simulink model "W05_2_idx_memory"  (R2024b)
settings: Solver=ode4  StartTime=0.0  StopTime=20  FixedStep=Ts_ctrl  RelTol=1e-3
values from neighbouring files (symbols this model uses):
  Ts_ctrl = 0.05    [W05_setup.m]    (also in W07_setup.m)
settings Model: Creator=admin  LastModifiedBy=admin

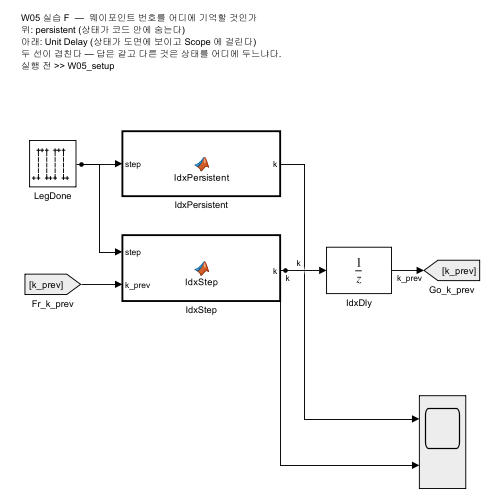
[thumbnail: Simulink's stored preview of the top-level diagram]
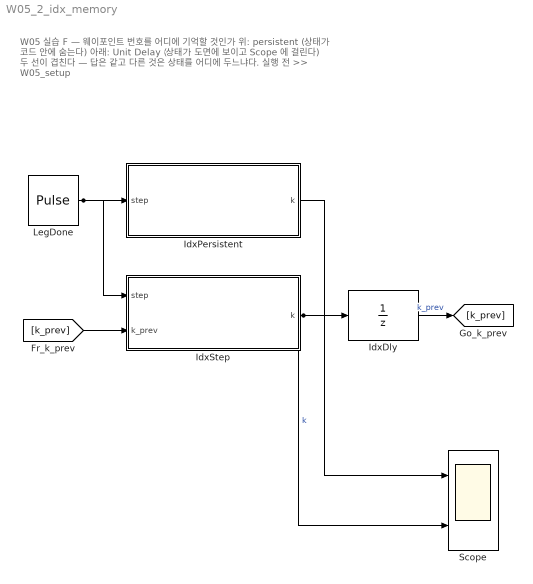
== system W05_2_idx_memory ==
  note: W05 실습 F  —  웨이포인트 번호를 어디에 기억할 것인가
      | 위: persistent (상태가 코드 안에 숨는다)
      | 아래: Unit Delay (상태가 도면에 보이고 Scope 에 걸린다)
      | 두 선이 겹친다 — 답은 같고 다른 것은 상태를 어디에 두느냐다.
      | 실행 전 >> W05_setup
  IdxDly : UnitDelay  Description=웨이포인트 번호의 기억. 정수 사건 상태이고 대수 루프를 끊는다 — 미분방정식의 상태가 아니므로 이산이 맞다.  InitialCondition=1  SampleTime=Ts_ctrl  HasFrameUpgradeWarning=on
  IdxPersistent : MATLAB Function  TreatAsAtomicUnit=on
  IdxStep : MATLAB Function  TreatAsAtomicUnit=on
  LegDone : DiscretePulseGenerator  Period=4/Ts_ctrl  SampleTime=Ts_ctrl
  Scope : Scope  NumInputPorts=2
  wires:
  LegDone/1 -> IdxPersistent/1(step), IdxStep/1(step)
  IdxStep/1(k) -> IdxDly/1, Scope/2  "k"
  IdxDly/1 -> [k_prev]  "k_prev"
  [k_prev] -> IdxStep/2(k_prev)
  IdxPersistent/1(k) -> Scope/1

== matlab function W05_2_idx_memory/IdxPersistent ==
  data: step input; k output
function k = IdxPersistent(step)
%#codegen
% 활성 웨이포인트 번호를 **함수 안에** 기억한다 (W05_matlab/LOSchi.m 방식).
% 상태가 코드 안에 숨어 도면에는 보이지 않는다.
persistent k_mem
if isempty(k_mem)
    k_mem = 1;
end
if step > 0.5
    k_mem = k_mem + 1;
end
k = k_mem;

== matlab function W05_2_idx_memory/IdxStep ==
  data: step input; k output; k_prev input
function k = IdxStep(step, k_prev)
%#codegen
% 기억하지 않는다 — **한 스텝 전의 값을 받아** 다음 값을 돌려줄 뿐이다.
% 기억은 밖의 Unit Delay 가 맡는다. 그래서 이 함수는 순수 함수다.
if step > 0.5
    k = k_prev + 1;
else
    k = k_prev;
end
